simulink model "WorkstationModel"  (Simulink 7.9)
settings: Solver=VariableStepDiscrete  StartTime=0.0  StopTime=100  RelTol=1e-3
settings Model: Creator=tsprock3  LastModifiedBy=tsprock3
settings DebuggingCC: SimStateOlderReleaseMsg=warning

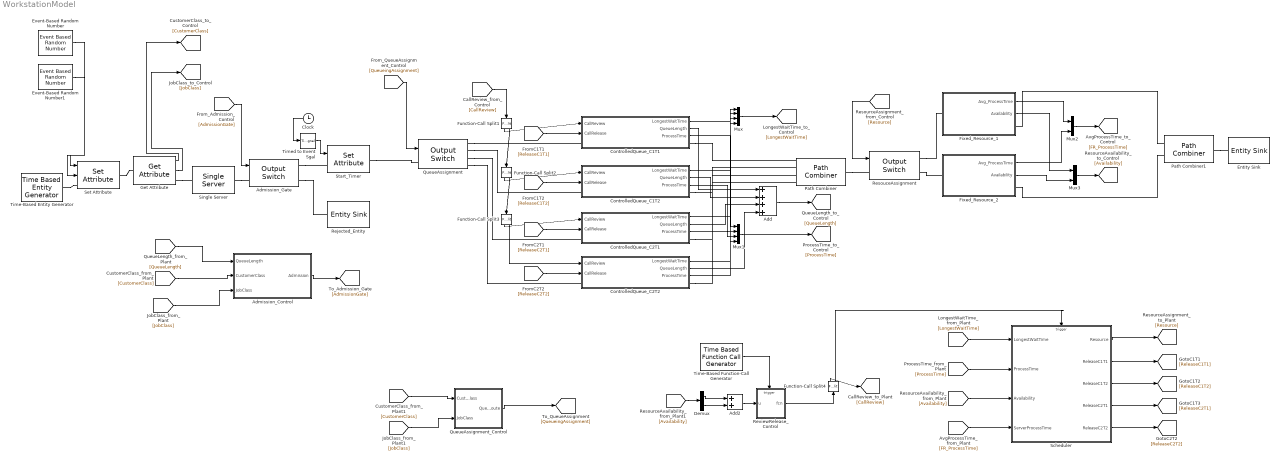
== system WorkstationModel ==
  Add : Sum  Inputs=++++
  Add2 : Sum
  Admission_Control : Truth Table  TreatAsAtomicUnit=on
  Admission_Gate : OutputSwitch  NumberOutputPorts=2  SwitchingCriterion=From signal port p
  Clock : Clock
  ControlledQueue_C1T1 : Subsystem
  ControlledQueue_C1T2 : Subsystem
  ControlledQueue_C2T1 : Subsystem
  ControlledQueue_C2T2 : Subsystem
  Demux : Demux  Outputs=2
  Entity Sink : EntitySink  StatNumberArrived=on
  Event-Based Random Number : EventBasedRandomNumber  Distribution=Arbitrary discrete  valueVecDisc=[1 2]  probVecDisc=[0.3 0.7]
  Event-Based Random Number1 : EventBasedRandomNumber  Distribution=Arbitrary discrete  valueVecDisc=[1 2]  probVecDisc=[.6 0.4]
  Fixed_Resource_1 : Subsystem
  Fixed_Resource_2 : Subsystem
  Function-Call Split{1..4} (4 alike) : FunctionCallSplit
  Get Attribute : GetAttribute  AttributeName=CustomerClass|JobClass  AttributeMissing=Error|Error  AttributeDefaultValue=1|1  AttributeTreatAsVector=1|1  AttributeSendTiming=After entity departure|After entity departure  EvaluatedDefaultAttributeValue={[];[]}
      settings: OutputPortMap=o1,o2
  Mux : Mux
  Mux1 : Mux
  Mux2 : Mux  Inputs=2
  Mux3 : Mux  Inputs=2
  Path Combiner : PathCombiner  NumberInputPorts=4
  Path Combiner1 : PathCombiner  NumberInputPorts=2
  QueueAssignment : OutputSwitch  NumberOutputPorts=4  SwitchingCriterion=From signal port p  EntityBufferOpt=on
  QueueAssignment_Control : Truth Table  TreatAsAtomicUnit=on
  Rejected_Entity : EntitySink
  ResouceAssignment : OutputSwitch  NumberOutputPorts=2  SwitchingCriterion=From signal port p  InitialConditionsOpt=on  EntityBufferOpt=on
  ReviewRelease_Control : Truth Table  TreatAsAtomicUnit=on
  Scheduler : MATLAB Function  TreatAsAtomicUnit=on
  Set Attribute : SetAttribute  AttributeName=CustomerClass|JobClass|ProcessTime  AttributeFrom=Signal port|Signal port|Dialog  AttributeValue=1|1|5  AttributeTreatAsVector=1|1|1  EvaluatedAttributeValue={[];[];5}
      settings: InputPortMap=u0,u1
  Single Server : SingleServer  ServiceTime=0
  Start_Timer : SetAttribute  AttributeName=EnterTime  AttributeFrom=Signal port  EvaluatedAttributeValue={[]}
  Time-Based Entity Generator : TimeBasedEntityGenerator  Period=9
  Time-Based Function-Call Generator : TimeBasedFunctionCallGenerator
  Timed to Event Sgal : TimedToEventSignal
  wires:
  ControlledQueue_C1T1/2(QueueLength) -> Add/1
  ControlledQueue_C1T2/2(QueueLength) -> Add/2
  ControlledQueue_C2T1/2(QueueLength) -> Add/3
  ControlledQueue_C2T2/2(QueueLength) -> Add/4
  Fixed_Resource_1/1(Avg_ProcessTime) -> Mux2/1
  Mux3/1 -> [Availability]
  Mux2/1 -> [FR_ProcessTime]
  Mux/1 -> [LongestWaitTime]
  ControlledQueue_C1T1/1(LongestWaitTime) -> Mux/1
  ControlledQueue_C1T2/1(LongestWaitTime) -> Mux/2
  ControlledQueue_C2T1/1(LongestWaitTime) -> Mux/3
  ControlledQueue_C2T2/1(LongestWaitTime) -> Mux/4
  Mux1/1 -> [ProcessTime]
  ControlledQueue_C1T1/3(ProcessTime) -> Mux1/1
  ControlledQueue_C1T2/3(ProcessTime) -> Mux1/2
  ControlledQueue_C2T1/3(ProcessTime) -> Mux1/3
  ControlledQueue_C2T2/3(ProcessTime) -> Mux1/4
  [Resource] -> ResouceAssignment/1
  Event-Based Random Number/1 -> Set Attribute/1
  Event-Based Random Number1/1 -> Set Attribute/2
  Timed to Event Sgal/1 -> Start_Timer/1
  Clock/1 -> Timed to Event Sgal/1
  Scheduler/1(Resource) -> [Resource]
  Function-Call Split4/2 -> Scheduler/Trigger
  [ProcessTime] -> Scheduler/2(ProcessTime)
  [LongestWaitTime] -> Scheduler/1(LongestWaitTime)
  Function-Call Split1/1 -> ControlledQueue_C1T1/1(CallReview)
  Function-Call Split1/2 -> Function-Call Split2/1
  Function-Call Split2/1 -> ControlledQueue_C1T2/1(CallReview)
  Function-Call Split2/2 -> Function-Call Split3/1
  Function-Call Split3/1 -> ControlledQueue_C2T1/1(CallReview)
  Function-Call Split3/2 -> ControlledQueue_C2T2/1(CallReview)
  Fixed_Resource_1/2(Availability) -> Mux3/1
  Fixed_Resource_2/2(Availability) -> Mux3/2
  Fixed_Resource_2/1(Avg_ProcessTime) -> Mux2/2
  Add2/1 -> ReviewRelease_Control/1(u)
  [Availability] -> Scheduler/3(Availability)
  [FR_ProcessTime] -> Scheduler/4(ServerProcessTime)
  Time-Based Function-Call Generator/1 -> ReviewRelease_Control/Trigger
  Scheduler/2(ReleaseC1T1) -> [ReleaseC1T1]
  Scheduler/3(ReleaseC1T2) -> [ReleaseC1T2]
  Scheduler/4(ReleaseC2T1) -> [ReleaseC2T1]
  Scheduler/5(ReleaseC2T2) -> [ReleaseC2T2]
  [ReleaseC1T1] -> ControlledQueue_C1T1/2(CallRelease)
  [ReleaseC1T2] -> ControlledQueue_C1T2/2(CallRelease)
  [ReleaseC2T1] -> ControlledQueue_C2T1/2(CallRelease)
  [ReleaseC2T2] -> ControlledQueue_C2T2/2(CallRelease)
  QueueAssignment_Control/1(QueueRoute) -> [QueueingAssignment]
  [QueueingAssignment] -> QueueAssignment/1
  Admission_Control/1(Admission) -> [AdmissionGate]
  [AdmissionGate] -> Admission_Gate/1
  Get Attribute/1 -> [CustomerClass]
  Get Attribute/2 -> [JobClass]
  [CustomerClass] -> Admission_Control/2(CustomerClass)
  [JobClass] -> Admission_Control/3(JobClass)
  [CustomerClass] -> QueueAssignment_Control/1(CustomerClass)
  [JobClass] -> QueueAssignment_Control/2(JobClass)
  Add/1 -> [QueueLength]
  [QueueLength] -> Admission_Control/1(QueueLength)
  [Availability] -> Demux/1
  Demux/1 -> Add2/1
  Demux/2 -> Add2/2
  [CallReview] -> Function-Call Split1/1
  Function-Call Split4/1 -> [CallReview]
  ReviewRelease_Control/1(fcn) -> Function-Call Split4/1
  connections:
  Fixed_Resource_1/RConn1 -- Path Combiner1/LConn1
  Admission_Gate/RConn1 -- Start_Timer/LConn1
  Single Server/RConn1 -- Admission_Gate/LConn1
  Get Attribute/RConn1 -- Single Server/LConn1
  Fixed_Resource_2/RConn1 -- Path Combiner1/LConn2
  Start_Timer/RConn1 -- QueueAssignment/LConn1
  QueueAssignment/RConn1 -- ControlledQueue_C1T1/LConn1
  QueueAssignment/RConn2 -- ControlledQueue_C1T2/LConn1
  QueueAssignment/RConn3 -- ControlledQueue_C2T1/LConn1
  QueueAssignment/RConn4 -- ControlledQueue_C2T2/LConn1
  ResouceAssignment/RConn1 -- Fixed_Resource_1/LConn1
  ResouceAssignment/RConn2 -- Fixed_Resource_2/LConn1
  Path Combiner/RConn1 -- ResouceAssignment/LConn1
  ControlledQueue_C1T1/RConn1 -- Path Combiner/LConn1
  ControlledQueue_C1T2/RConn1 -- Path Combiner/LConn2
  ControlledQueue_C2T1/RConn1 -- Path Combiner/LConn3
  ControlledQueue_C2T2/RConn1 -- Path Combiner/LConn4
  Path Combiner1/RConn1 -- Entity Sink/LConn1
  Time-Based Entity Generator/RConn1 -- Set Attribute/LConn1
  Set Attribute/RConn1 -- Get Attribute/LConn1
  Admission_Gate/RConn2 -- Rejected_Entity/LConn1

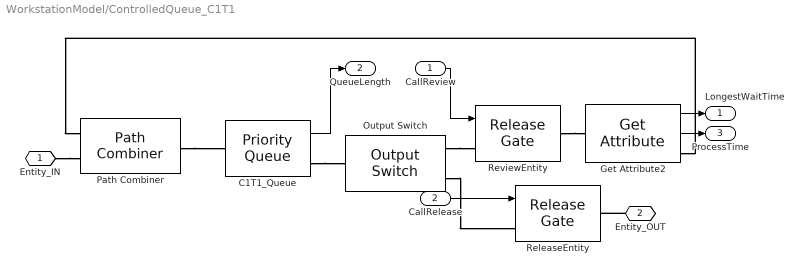
== system WorkstationModel/ControlledQueue_C1T1 ==
  CallReview : Inport
  CallRelease : Inport  Port=2
  C1T1_Queue : PriorityQueue  Capacity=inf  SortingAttributeName=EnterTime  StatNumberInBlock=on
      settings: OutputPortMap=o1
  Get Attribute2 : GetAttribute  AttributeName=EnterTime|ProcessTime  AttributeMissing=Error|Error  AttributeDefaultValue=1|1  AttributeTreatAsVector=1|1  AttributeSendTiming=After entity departure|After entity departure  EvaluatedDefaultAttributeValue={[];[]}
      settings: OutputPortMap=o1,o2
  Output Switch : OutputSwitch  NumberOutputPorts=2
  Path Combiner : PathCombiner  NumberInputPorts=2
  ReleaseEntity : ReleaseGate  OpenGateUpon=Function call from port fcn
  ReviewEntity : ReleaseGate  OpenGateUpon=Function call from port fcn
  Entity_IN : PMIOPort  Port=1  Side=Left
  Entity_OUT : PMIOPort  Port=2  Side=Right
  LongestWaitTime : Outport
  QueueLength : Outport  Port=2
  ProcessTime : Outport  Port=3
  wires:
  Get Attribute2/1 -> LongestWaitTime/1
  CallReview/1 -> ReviewEntity/1
  C1T1_Queue/1 -> QueueLength/1
  Get Attribute2/2 -> ProcessTime/1
  CallRelease/1 -> ReleaseEntity/1
  connections:
  Path Combiner/RConn1 -- C1T1_Queue/LConn1
  C1T1_Queue/RConn1 -- Output Switch/LConn1
  ReviewEntity/RConn1 -- Get Attribute2/LConn1
  Get Attribute2/RConn1 -- Path Combiner/LConn1
  Output Switch/RConn1 -- ReviewEntity/LConn1
  Output Switch/RConn2 -- ReleaseEntity/LConn1
  Entity_IN/RConn1 -- Path Combiner/LConn2
  Entity_OUT/RConn1 -- ReleaseEntity/RConn1

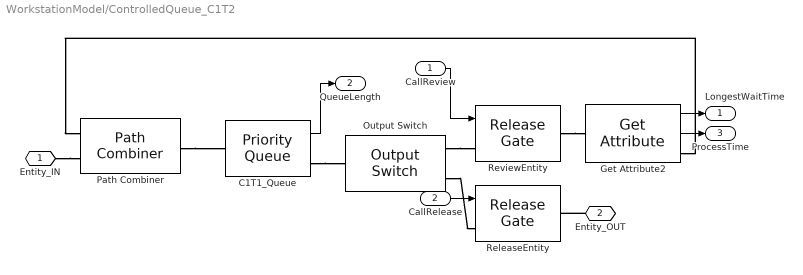
== system WorkstationModel/ControlledQueue_C1T2 ==
  CallReview : Inport
  CallRelease : Inport  Port=2
  C1T1_Queue : PriorityQueue  Capacity=inf  SortingAttributeName=EnterTime  StatNumberInBlock=on
      settings: OutputPortMap=o1
  Get Attribute2 : GetAttribute  AttributeName=EnterTime|ProcessTime  AttributeMissing=Error|Error  AttributeDefaultValue=1|1  AttributeTreatAsVector=1|1  AttributeSendTiming=After entity departure|After entity departure  EvaluatedDefaultAttributeValue={[];[]}
      settings: OutputPortMap=o1,o2
  Output Switch : OutputSwitch  NumberOutputPorts=2
  Path Combiner : PathCombiner  NumberInputPorts=2
  ReleaseEntity : ReleaseGate  OpenGateUpon=Function call from port fcn
  ReviewEntity : ReleaseGate  OpenGateUpon=Function call from port fcn
  Entity_IN : PMIOPort  Port=1  Side=Left
  Entity_OUT : PMIOPort  Port=2  Side=Right
  LongestWaitTime : Outport
  QueueLength : Outport  Port=2
  ProcessTime : Outport  Port=3
  wires:
  Get Attribute2/1 -> LongestWaitTime/1
  CallReview/1 -> ReviewEntity/1
  C1T1_Queue/1 -> QueueLength/1
  Get Attribute2/2 -> ProcessTime/1
  CallRelease/1 -> ReleaseEntity/1
  connections:
  Path Combiner/RConn1 -- C1T1_Queue/LConn1
  C1T1_Queue/RConn1 -- Output Switch/LConn1
  ReviewEntity/RConn1 -- Get Attribute2/LConn1
  Get Attribute2/RConn1 -- Path Combiner/LConn1
  Output Switch/RConn1 -- ReviewEntity/LConn1
  Output Switch/RConn2 -- ReleaseEntity/LConn1
  Entity_IN/RConn1 -- Path Combiner/LConn2
  Entity_OUT/RConn1 -- ReleaseEntity/RConn1

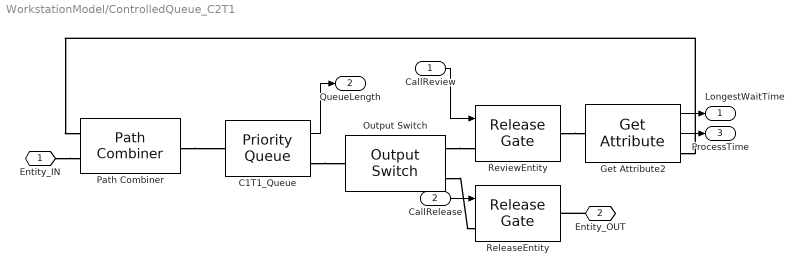
== system WorkstationModel/ControlledQueue_C2T1 ==
  CallReview : Inport
  CallRelease : Inport  Port=2
  C1T1_Queue : PriorityQueue  Capacity=inf  SortingAttributeName=EnterTime  StatNumberInBlock=on
      settings: OutputPortMap=o1
  Get Attribute2 : GetAttribute  AttributeName=EnterTime|ProcessTime  AttributeMissing=Error|Error  AttributeDefaultValue=1|1  AttributeTreatAsVector=1|1  AttributeSendTiming=After entity departure|After entity departure  EvaluatedDefaultAttributeValue={[];[]}
      settings: OutputPortMap=o1,o2
  Output Switch : OutputSwitch  NumberOutputPorts=2
  Path Combiner : PathCombiner  NumberInputPorts=2
  ReleaseEntity : ReleaseGate  OpenGateUpon=Function call from port fcn
  ReviewEntity : ReleaseGate  OpenGateUpon=Function call from port fcn
  Entity_IN : PMIOPort  Port=1  Side=Left
  Entity_OUT : PMIOPort  Port=2  Side=Right
  LongestWaitTime : Outport
  QueueLength : Outport  Port=2
  ProcessTime : Outport  Port=3
  wires:
  Get Attribute2/1 -> LongestWaitTime/1
  CallReview/1 -> ReviewEntity/1
  C1T1_Queue/1 -> QueueLength/1
  Get Attribute2/2 -> ProcessTime/1
  CallRelease/1 -> ReleaseEntity/1
  connections:
  Path Combiner/RConn1 -- C1T1_Queue/LConn1
  C1T1_Queue/RConn1 -- Output Switch/LConn1
  ReviewEntity/RConn1 -- Get Attribute2/LConn1
  Get Attribute2/RConn1 -- Path Combiner/LConn1
  Output Switch/RConn1 -- ReviewEntity/LConn1
  Output Switch/RConn2 -- ReleaseEntity/LConn1
  Entity_IN/RConn1 -- Path Combiner/LConn2
  Entity_OUT/RConn1 -- ReleaseEntity/RConn1

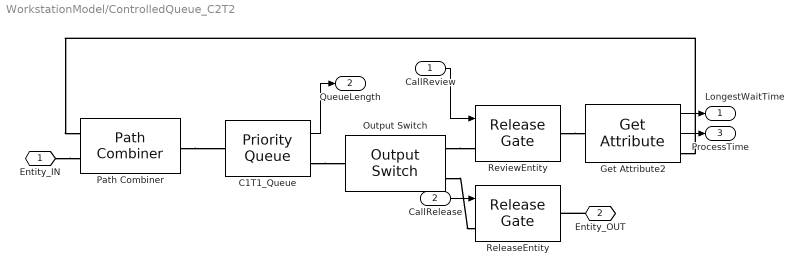
== system WorkstationModel/ControlledQueue_C2T2 ==
  CallReview : Inport
  CallRelease : Inport  Port=2
  C1T1_Queue : PriorityQueue  Capacity=inf  SortingAttributeName=EnterTime  StatNumberInBlock=on
      settings: OutputPortMap=o1
  Get Attribute2 : GetAttribute  AttributeName=EnterTime|ProcessTime  AttributeMissing=Error|Error  AttributeDefaultValue=1|1  AttributeTreatAsVector=1|1  AttributeSendTiming=After entity departure|After entity departure  EvaluatedDefaultAttributeValue={[];[]}
      settings: OutputPortMap=o1,o2
  Output Switch : OutputSwitch  NumberOutputPorts=2
  Path Combiner : PathCombiner  NumberInputPorts=2
  ReleaseEntity : ReleaseGate  OpenGateUpon=Function call from port fcn
  ReviewEntity : ReleaseGate  OpenGateUpon=Function call from port fcn
  Entity_IN : PMIOPort  Port=1  Side=Left
  Entity_OUT : PMIOPort  Port=2  Side=Right
  LongestWaitTime : Outport
  QueueLength : Outport  Port=2
  ProcessTime : Outport  Port=3
  wires:
  Get Attribute2/1 -> LongestWaitTime/1
  CallReview/1 -> ReviewEntity/1
  C1T1_Queue/1 -> QueueLength/1
  Get Attribute2/2 -> ProcessTime/1
  CallRelease/1 -> ReleaseEntity/1
  connections:
  Path Combiner/RConn1 -- C1T1_Queue/LConn1
  C1T1_Queue/RConn1 -- Output Switch/LConn1
  ReviewEntity/RConn1 -- Get Attribute2/LConn1
  Get Attribute2/RConn1 -- Path Combiner/LConn1
  Output Switch/RConn1 -- ReviewEntity/LConn1
  Output Switch/RConn2 -- ReleaseEntity/LConn1
  Entity_IN/RConn1 -- Path Combiner/LConn2
  Entity_OUT/RConn1 -- ReleaseEntity/RConn1

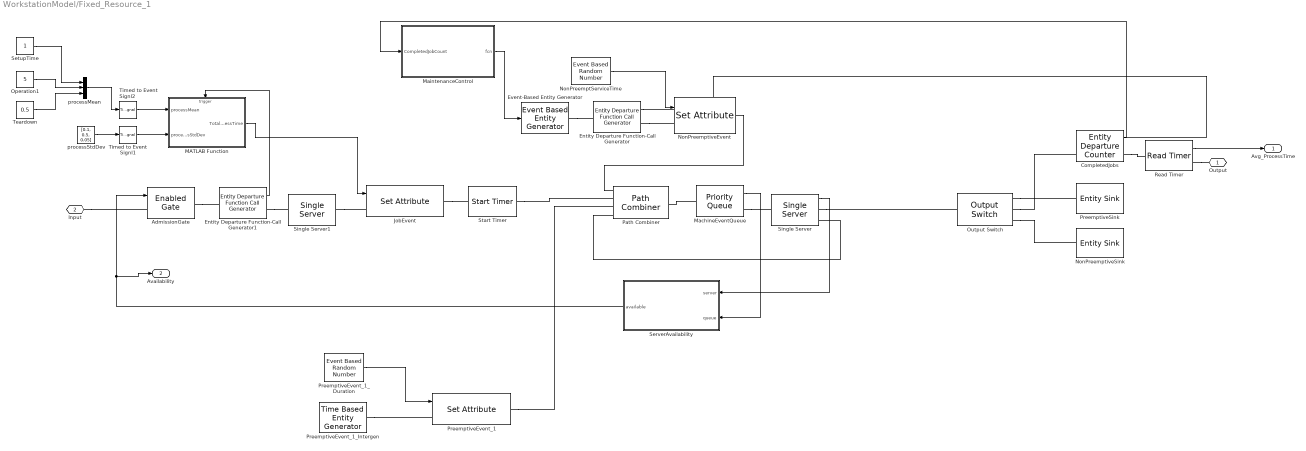
== system WorkstationModel/Fixed_Resource_1 ==
  AdmissionGate : EnabledGate
  CompletedJobs : EntityDepartureCounter  NumberDepartedToSignal=on  NumberDepartedToAttribute=off  CounterResetTypeOption=Function call from port fcn  SpecifyEventPriority=on
  Entity Departure Function-Call Generator : EntityDepartureFunctionCallGenerator
  Entity Departure Function-Call Generator1 : EntityDepartureFunctionCallGenerator
  Event-Based Entity Generator : EventBasedEntityGenerator  GenerateEntitiesUpon=Function call from port fcn  GenerateEntityAtSimulationStart=off
  JobEvent : SetAttribute  AttributeName=ServiceTime|PreemptiveEventClass  AttributeFrom=Signal port|Dialog  AttributeValue=1|2  AttributeTreatAsVector=1|1  EvaluatedAttributeValue={[];2}
  MATLAB Function : MATLAB Function  TreatAsAtomicUnit=on
  MachineEventQueue : PriorityQueue  Capacity=inf  SortingAttributeName=PreemptiveEventClass  StatNumberInBlock=on
      settings: OutputPortMap=o1
  MaintenanceControl : Truth Table  TreatAsAtomicUnit=on
  NonPreemptServiceTime : EventBasedRandomNumber  Seed=27991
  NonPreemptiveEvent : SetAttribute  AttributeName=ServiceTime|PreemptiveEventClass  AttributeFrom=Signal port|Dialog  AttributeValue=1|3  AttributeTreatAsVector=1|1  EvaluatedAttributeValue={[];3}
  NonPreemptiveSink : EntitySink
  Operation1 : Constant  Value=5
  Output Switch : OutputSwitch  SwitchingCriterion=From attribute  AttributeName=PreemptiveEventClass
  Path Combiner : PathCombiner  NumberInputPorts=4
  PreemptiveEvent_1 : SetAttribute  AttributeName=ServiceTime|PreemptiveEventClass  AttributeFrom=Signal port|Dialog  AttributeValue=1|1  AttributeTreatAsVector=1|1  EvaluatedAttributeValue={[];1}
  PreemptiveEvent_1_Duration : EventBasedRandomNumber  meanExp=3
  PreemptiveEvent_1_Intergen : TimeBasedEntityGenerator  Period=100  GenerateEntityAtSimulationStart=off
  PreemptiveSink : EntitySink
  Read Timer : ReadTimer  StatAverageTimeElapsed=on
      settings: OutputPortMap=o3
  ServerAvailability : Truth Table  TreatAsAtomicUnit=on
  SetupTime : Constant
  Single Server : SingleServer  ServiceTimeFrom=Attribute  PermitPreemption=on  SortingAttributeName=PreemptiveEventClass  WriteToAttribute=on  ResidualAttributeName=ServiceTime  StatNumberInBlock=on
      settings: OutputPortMap=o1
  Single Server1 : SingleServer  ServiceTime=0
  Start Timer : StartTimer
  Teardown : Constant  Value=0.5
  Timed to Event Signl1 : TimedToEventSignal
  Timed to Event Signl2 : TimedToEventSignal
  processMean : Concatenate  NumInputs=3
  processStdDev : Constant  Value=[0.1, 0.5, 0.05]
  Output : PMIOPort  Port=1  Side=Right
  Input : PMIOPort  Port=2  Side=Left
  Avg_ProcessTime : Outport
  Availability : Outport  Port=2
  wires:
  PreemptiveEvent_1_Duration/1 -> PreemptiveEvent_1/1
  CompletedJobs/1 -> MaintenanceControl/1(CompletedJobCount)
  NonPreemptServiceTime/1 -> NonPreemptiveEvent/1
  ServerAvailability/1(available) -> AdmissionGate/1, Availability/1
  MachineEventQueue/1 -> ServerAvailability/2(queue)
  Single Server/1 -> ServerAvailability/1(server)
  MaintenanceControl/1(fcn) -> Event-Based Entity Generator/1
  MATLAB Function/1(TotalProcessTime) -> JobEvent/1
  Entity Departure Function-Call Generator/1 -> CompletedJobs/1
  Entity Departure Function-Call Generator1/1 -> MATLAB Function/Trigger
  processStdDev/1 -> Timed to Event Signl1/1
  Timed to Event Signl1/1 -> MATLAB Function/2(processStdDev)
  Timed to Event Signl2/1 -> MATLAB Function/1(processMean)
  processMean/1 -> Timed to Event Signl2/1
  Teardown/1 -> processMean/3
  Operation1/1 -> processMean/2
  SetupTime/1 -> processMean/1
  Read Timer/1 -> Avg_ProcessTime/1
  connections:
  PreemptiveEvent_1_Intergen/RConn1 -- PreemptiveEvent_1/LConn1
  MachineEventQueue/RConn1 -- Single Server/LConn1
  Path Combiner/RConn1 -- MachineEventQueue/LConn1
  Output Switch/RConn3 -- NonPreemptiveSink/LConn1
  Output Switch/RConn1 -- PreemptiveSink/LConn1
  Path Combiner/LConn4 -- Single Server/RConn2
  PreemptiveEvent_1/RConn1 -- Path Combiner/LConn3
  Output Switch/RConn2 -- CompletedJobs/LConn1
  NonPreemptiveEvent/RConn1 -- Path Combiner/LConn1
  Input/RConn1 -- AdmissionGate/LConn1
  Event-Based Entity Generator/RConn1 -- Entity Departure Function-Call Generator/LConn1
  Entity Departure Function-Call Generator/RConn1 -- NonPreemptiveEvent/LConn1
  AdmissionGate/RConn1 -- Entity Departure Function-Call Generator1/LConn1
  Entity Departure Function-Call Generator1/RConn1 -- Single Server1/LConn1
  Single Server1/RConn1 -- JobEvent/LConn1
  JobEvent/RConn1 -- Start Timer/LConn1
  Start Timer/RConn1 -- Path Combiner/LConn2
  CompletedJobs/RConn1 -- Read Timer/LConn1
  Read Timer/RConn1 -- Output/RConn1
  Single Server/RConn1 -- Output Switch/LConn1

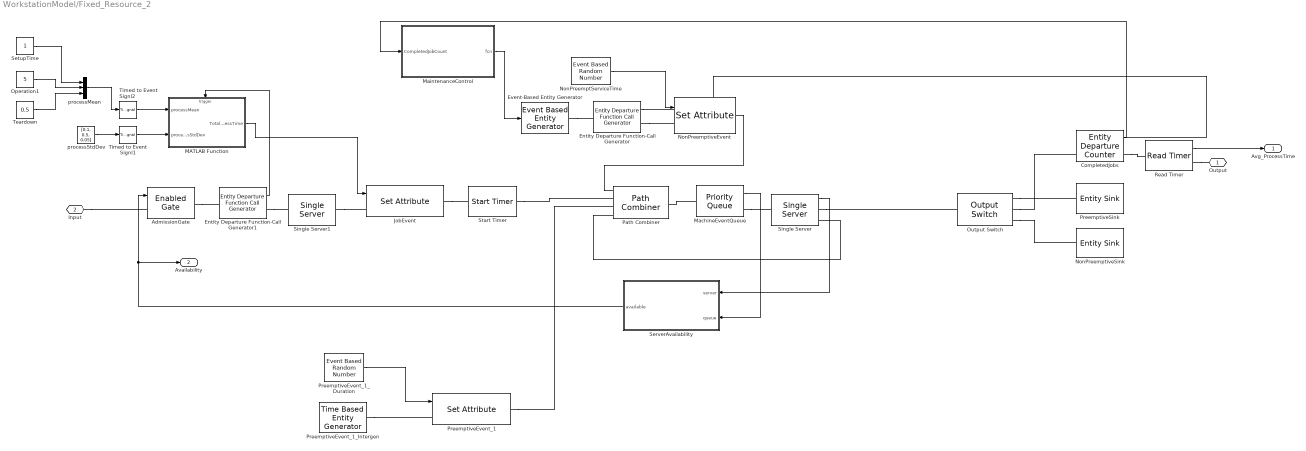
== system WorkstationModel/Fixed_Resource_2 ==
  AdmissionGate : EnabledGate
  CompletedJobs : EntityDepartureCounter  NumberDepartedToSignal=on  NumberDepartedToAttribute=off  CounterResetTypeOption=Function call from port fcn  SpecifyEventPriority=on
  Entity Departure Function-Call Generator : EntityDepartureFunctionCallGenerator
  Entity Departure Function-Call Generator1 : EntityDepartureFunctionCallGenerator
  Event-Based Entity Generator : EventBasedEntityGenerator  GenerateEntitiesUpon=Function call from port fcn  GenerateEntityAtSimulationStart=off
  JobEvent : SetAttribute  AttributeName=ServiceTime|PreemptiveEventClass  AttributeFrom=Signal port|Dialog  AttributeValue=1|2  AttributeTreatAsVector=1|1  EvaluatedAttributeValue={[];2}
  MATLAB Function : MATLAB Function  TreatAsAtomicUnit=on
  MachineEventQueue : PriorityQueue  Capacity=inf  SortingAttributeName=PreemptiveEventClass  StatNumberInBlock=on
      settings: OutputPortMap=o1
  MaintenanceControl : Truth Table  TreatAsAtomicUnit=on
  NonPreemptServiceTime : EventBasedRandomNumber  Seed=27991
  NonPreemptiveEvent : SetAttribute  AttributeName=ServiceTime|PreemptiveEventClass  AttributeFrom=Signal port|Dialog  AttributeValue=1|3  AttributeTreatAsVector=1|1  EvaluatedAttributeValue={[];3}
  NonPreemptiveSink : EntitySink
  Operation1 : Constant  Value=5
  Output Switch : OutputSwitch  SwitchingCriterion=From attribute  AttributeName=PreemptiveEventClass
  Path Combiner : PathCombiner  NumberInputPorts=4
  PreemptiveEvent_1 : SetAttribute  AttributeName=ServiceTime|PreemptiveEventClass  AttributeFrom=Signal port|Dialog  AttributeValue=1|1  AttributeTreatAsVector=1|1  EvaluatedAttributeValue={[];1}
  PreemptiveEvent_1_Duration : EventBasedRandomNumber  meanExp=3
  PreemptiveEvent_1_Intergen : TimeBasedEntityGenerator  Period=100  GenerateEntityAtSimulationStart=off
  PreemptiveSink : EntitySink
  Read Timer : ReadTimer  StatAverageTimeElapsed=on
      settings: OutputPortMap=o3
  ServerAvailability : Truth Table  TreatAsAtomicUnit=on
  SetupTime : Constant
  Single Server : SingleServer  ServiceTimeFrom=Attribute  PermitPreemption=on  SortingAttributeName=PreemptiveEventClass  WriteToAttribute=on  ResidualAttributeName=ServiceTime  StatNumberInBlock=on
      settings: OutputPortMap=o1
  Single Server1 : SingleServer  ServiceTime=0
  Start Timer : StartTimer
  Teardown : Constant  Value=0.5
  Timed to Event Signl1 : TimedToEventSignal
  Timed to Event Signl2 : TimedToEventSignal
  processMean : Concatenate  NumInputs=3
  processStdDev : Constant  Value=[0.1, 0.5, 0.05]
  Output : PMIOPort  Port=1  Side=Right
  Input : PMIOPort  Port=2  Side=Left
  Avg_ProcessTime : Outport
  Availability : Outport  Port=2
  wires:
  PreemptiveEvent_1_Duration/1 -> PreemptiveEvent_1/1
  CompletedJobs/1 -> MaintenanceControl/1(CompletedJobCount)
  NonPreemptServiceTime/1 -> NonPreemptiveEvent/1
  ServerAvailability/1(available) -> AdmissionGate/1, Availability/1
  MachineEventQueue/1 -> ServerAvailability/2(queue)
  Single Server/1 -> ServerAvailability/1(server)
  MaintenanceControl/1(fcn) -> Event-Based Entity Generator/1
  MATLAB Function/1(TotalProcessTime) -> JobEvent/1
  Entity Departure Function-Call Generator/1 -> CompletedJobs/1
  Entity Departure Function-Call Generator1/1 -> MATLAB Function/Trigger
  processStdDev/1 -> Timed to Event Signl1/1
  Timed to Event Signl1/1 -> MATLAB Function/2(processStdDev)
  Timed to Event Signl2/1 -> MATLAB Function/1(processMean)
  processMean/1 -> Timed to Event Signl2/1
  Teardown/1 -> processMean/3
  Operation1/1 -> processMean/2
  SetupTime/1 -> processMean/1
  Read Timer/1 -> Avg_ProcessTime/1
  connections:
  PreemptiveEvent_1_Intergen/RConn1 -- PreemptiveEvent_1/LConn1
  MachineEventQueue/RConn1 -- Single Server/LConn1
  Path Combiner/RConn1 -- MachineEventQueue/LConn1
  Output Switch/RConn3 -- NonPreemptiveSink/LConn1
  Output Switch/RConn1 -- PreemptiveSink/LConn1
  Path Combiner/LConn4 -- Single Server/RConn2
  PreemptiveEvent_1/RConn1 -- Path Combiner/LConn3
  Output Switch/RConn2 -- CompletedJobs/LConn1
  NonPreemptiveEvent/RConn1 -- Path Combiner/LConn1
  Input/RConn1 -- AdmissionGate/LConn1
  Event-Based Entity Generator/RConn1 -- Entity Departure Function-Call Generator/LConn1
  Entity Departure Function-Call Generator/RConn1 -- NonPreemptiveEvent/LConn1
  AdmissionGate/RConn1 -- Entity Departure Function-Call Generator1/LConn1
  Entity Departure Function-Call Generator1/RConn1 -- Single Server1/LConn1
  Single Server1/RConn1 -- JobEvent/LConn1
  JobEvent/RConn1 -- Start Timer/LConn1
  Start Timer/RConn1 -- Path Combiner/LConn2
  CompletedJobs/RConn1 -- Read Timer/LConn1
  Read Timer/RConn1 -- Output/RConn1
  Single Server/RConn1 -- Output Switch/LConn1

== matlab function Admission_Control ==
  data: QueueLength input double; Admission output double; CustomerClass input double; JobClass input double
function Admission = fcn(QueueLength, CustomerClass, JobClass)

aVarTruthTableCondition_1 = false;
aVarTruthTableCondition_2 = false;


% Short Queue

aVarTruthTableCondition_1 = logical(QueueLength < 10);

% Priority Customer

aVarTruthTableCondition_2 = logical(CustomerClass == 1);

if (aVarTruthTableCondition_1 && aVarTruthTableCondition_2)
    aFcnTruthTableAction_1();
elseif (aVarTruthTableCondition_1 && ~aVarTruthTableCondition_2)
    aFcnTruthTableAction_1();
elseif (~aVarTruthTableCondition_1 && aVarTruthTableCondition_2)
    aFcnTruthTableAction_1();
else % Default
    aFcnTruthTableAction_2();
end

function aFcnTruthTableAction_1()

% Example action 1 called from D1 & D2 column in condition table

Admission = 1;

function aFcnTruthTableAction_2()

% Example action 2 called from D3 column in condition table

Admission = 2;

== matlab function Fixed_Resource_1/MATLAB Function ==
  data: TotalProcessTime output double; processMean input double; processStdDev input double
  events: Arrival input FUNCTION_CALL_EVENT
function TotalProcessTime = fcn(processMean, processStdDev)
%#codegen

coder.extrinsic('normrnd');
TotalProcessTime = zeros(1,'double');

TotalProcessTime = sum(normrnd(processMean, processStdDev));

== matlab function Fixed_Resource_1/MaintenanceControl ==
  data: CompletedJobCount input double
  events: fcn output FUNCTION_CALL_EVENT
function fcn(CompletedJobCount)

aVarTruthTableCondition_1 = false;


% NonPreemptive Maintenance

aVarTruthTableCondition_1 = logical(CompletedJobCount == 10);

if (aVarTruthTableCondition_1)
    aFcnTruthTableAction_1();
else % Default
    aFcnTruthTableAction_2();
end

function aFcnTruthTableAction_1()

% Create Maintenance Job

fcn;

function aFcnTruthTableAction_2()

% Do Nothing

== matlab function Fixed_Resource_1/ServerAvailability ==
  data: server input double; available output double; queue input double
function available = fcn(server, queue)

aVarTruthTableCondition_1 = false;
aVarTruthTableCondition_2 = false;


% Server Busy

aVarTruthTableCondition_1 = logical(server > 0);

% Preemptive Events Waiting

aVarTruthTableCondition_2 = logical(queue > 0);

if (aVarTruthTableCondition_1 && aVarTruthTableCondition_2)
    aFcnTruthTableAction_1();
elseif (aVarTruthTableCondition_1 && ~aVarTruthTableCondition_2)
    aFcnTruthTableAction_1();
elseif (~aVarTruthTableCondition_1 && aVarTruthTableCondition_2)
    aFcnTruthTableAction_1();
else % Default
    aFcnTruthTableAction_2();
end

function aFcnTruthTableAction_1()

% Machine Unavailable

available = 0;

function aFcnTruthTableAction_2()

% Machine Available

available = 1;

== matlab function ReviewRelease_Control ==
  data: u input double
  events: fcn output FUNCTION_CALL_EVENT; trigger input FUNCTION_CALL_EVENT
function fcn(u)

aVarTruthTableCondition_1 = false;


% Example condition 1

aVarTruthTableCondition_1 = logical(u > 0);

if (aVarTruthTableCondition_1)
    aFcnTruthTableAction_1();
else % Default
    aFcnTruthTableAction_2();
end

function aFcnTruthTableAction_1()

% function call.

fcn;

function aFcnTruthTableAction_2()

% do nothing

== matlab function Fixed_Resource_2/MATLAB Function ==
  data: TotalProcessTime output double; processMean input double; processStdDev input double
  events: Arrival input FUNCTION_CALL_EVENT
function TotalProcessTime = fcn(processMean, processStdDev)
%#codegen

coder.extrinsic('normrnd');
TotalProcessTime = zeros(1,'double');

TotalProcessTime = sum(normrnd(processMean, processStdDev));

== matlab function Fixed_Resource_2/MaintenanceControl ==
  data: CompletedJobCount input double
  events: fcn output FUNCTION_CALL_EVENT
function fcn(CompletedJobCount)

aVarTruthTableCondition_1 = false;


% NonPreemptive Maintenance

aVarTruthTableCondition_1 = logical(CompletedJobCount == 10);

if (aVarTruthTableCondition_1)
    aFcnTruthTableAction_1();
else % Default
    aFcnTruthTableAction_2();
end

function aFcnTruthTableAction_1()

% Create Maintenance Job

fcn;

function aFcnTruthTableAction_2()

% Do Nothing

== matlab function QueueAssignment_Control ==
  data: CustomerClass input double; QueueRoute output double; JobClass input double
function QueueRoute = fcn(CustomerClass, JobClass)

aVarTruthTableCondition_1 = false;
aVarTruthTableCondition_2 = false;


% CustomerClass

aVarTruthTableCondition_1 = logical(CustomerClass==1);

% JobClass

aVarTruthTableCondition_2 = logical(JobClass==1);

if (aVarTruthTableCondition_1 && aVarTruthTableCondition_2)
    aFcnTruthTableAction_1();
elseif (aVarTruthTableCondition_1 && ~aVarTruthTableCondition_2)
    aFcnTruthTableAction_2();
elseif (~aVarTruthTableCondition_1 && aVarTruthTableCondition_2)
    aFcnTruthTableAction_3();
else % Default
    aFcnTruthTableAction_4();
end

function aFcnTruthTableAction_1()

% C1T1

QueueRoute = 1;

function aFcnTruthTableAction_2()

% C1T2

QueueRoute = 2;

function aFcnTruthTableAction_3()

% C2T1

QueueRoute = 3;

function aFcnTruthTableAction_4()

% C2T2

QueueRoute = 4;

== matlab function Scheduler ==
  data: LongestWaitTime input double; ProcessTime input double; Availability input double; ServerProcessTime input double; Resource output double
  events: ServerAvailable input FUNCTION_CALL_EVENT; ReleaseC1T1 output FUNCTION_CALL_EVENT; ReleaseC1T2 output FUNCTION_CALL_EVENT; ReleaseC2T1 output FUNCTION_CALL_EVENT; ReleaseC2T2 output FUNCTION_CALL_EVENT
function Resource  = fcn(LongestWaitTime, ProcessTime, Availability, ServerProcessTime)
%#codegen


NZ = find(ProcessTime);
%Release = [0 0 0 0];
Resource = 1;

if isempty(NZ) ==0
    quotedleadtime = [14 21 21 28]'; %[C1T1 C1T2 C2T1 C2T2]

    TotalDelay = LongestWaitTime + ProcessTime;

    TotalPenalty = [3 3 6 6]'./(TotalDelay - quotedleadtime).^2;

    %Release job based on max penalty cost
    [Y, I] = max(TotalPenalty(NZ));

    %Release(NZ(I(1))) = 1;

    %If Resource Available
    if isempty(find(Availability, 1)) == 0
        %Assign Resource
        if Availability(1) ==1
            Resource = 1;
        elseif Availability(2) ==1
            Resource = 2;
        end
        
        
        %Release a Job from a Queue
        switch NZ(I(1))
            case 1
                ReleaseC1T1;
            case 2
                ReleaseC1T2;
            case 3
                ReleaseC2T1;
            case 4
                ReleaseC2T2;
        end
    end

end

== matlab function Fixed_Resource_2/ServerAvailability ==
  data: server input double; available output double; queue input double
function available = fcn(server, queue)

aVarTruthTableCondition_1 = false;
aVarTruthTableCondition_2 = false;


% Server Busy

aVarTruthTableCondition_1 = logical(server > 0);

% Preemptive Events Waiting

aVarTruthTableCondition_2 = logical(queue > 0);

if (aVarTruthTableCondition_1 && aVarTruthTableCondition_2)
    aFcnTruthTableAction_1();
elseif (aVarTruthTableCondition_1 && ~aVarTruthTableCondition_2)
    aFcnTruthTableAction_1();
elseif (~aVarTruthTableCondition_1 && aVarTruthTableCondition_2)
    aFcnTruthTableAction_1();
else % Default
    aFcnTruthTableAction_2();
end

function aFcnTruthTableAction_1()

% Machine Unavailable

available = 0;

function aFcnTruthTableAction_2()

% Machine Available

available = 1;
